simulink model "sim_cv3"  (R2019b)
settings: Solver=FixedStepAuto  StartTime=0.0  StopTime=1040  FixedStep=1  RelTol=1e-3
values from neighbouring files (symbols this model uses):
  AG = 0.95    [identifikacia_simulatora.m]    (also in identifikacia_simulatora2.m; simulator.m)
  G_INIT = 153    [cv5.m]    (also in identifikacia_simulatora.m = 158.4; identifikacia_simulatora2.m; simulator.m)
  GB = G_INIT    (= 158.4)    [identifikacia_simulatora.m]    (also in identifikacia_simulatora2.m = 153; simulator.m = 153)
  kI = ki    (= 0.1645)    [identifikacia_simulatora.m]    (also in identifikacia_simulatora2.m = 0.1939; simulator.m)
  p2 = 0.0106    [cv5.m]    (also in identifikacia_simulatora.m; identifikacia_simulatora2.m = 0.0097; simulator.m)
  p3 = p2    (= 0.0097)    [identifikacia_simulatora2.m]
  SG = S_G    (= 0.032)    [identifikacia_simulatora.m]    (also in identifikacia_simulatora2.m = 0.0159; simulator.m)
  SI = S_I    (= 0.00159)    [identifikacia_simulatora.m]    (also in identifikacia_simulatora2.m = 0.0014; simulator.m)
  TD = 33.474    [identifikacia_simulatora.m]    (also in identifikacia_simulatora2.m = 41.1727; simulator.m)
  TI = 44.55    [cv5.m]    (also in identifikacia_simulatora.m; identifikacia_simulatora2.m = 42.8216; simulator.m)
  VG = V_G    (= 1.467)    [identifikacia_simulatora.m]    (also in identifikacia_simulatora2.m; simulator.m)
  VI = 138.8    [cv5.m]    (also in identifikacia_simulatora.m; identifikacia_simulatora2.m = 110.599; simulator.m)
undefined symbols (not defined in the file or in its folder): p22, sigbuilder_block
settings Model: Creator=Miroslava  LastModifiedBy=shneeder
settings DataIOCC: ReturnWorkspaceOutputs=off
settings DebuggingCC: ArithmeticOperatorsInVariantConditions=warning
settings SFSimCC: SimUseLocalCustomCode=off  CustomCodeUndefinedFunction=UseInterfaceOnly
settings RTWCC: RTWUseLocalCustomCode=off

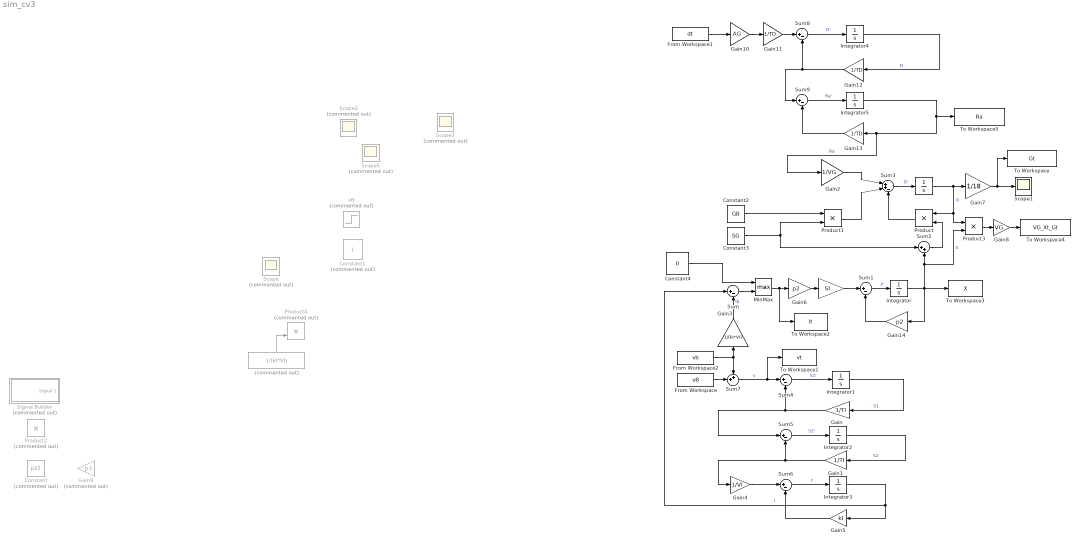
== system sim_cv3 ==
  " " : Gain  Gain=SI
  "   " : Integrator  InitialCondition=G_INIT
  " " : Constant  Commented=on  Value=1/(kI*VI)
  Constant : Constant  Commented=on  Value=p22
  Constant1 : Constant  Commented=on
  Constant2 : Constant  Value=GB
  Constant3 : Constant  Value=SG
  Constant4 : Constant  Value=0
  From Workspace : FromWorkspace  VariableName=vB  SampleTime=0
  From Workspace1 : FromWorkspace  VariableName=dt  SampleTime=0
  From Workspace2 : FromWorkspace  VariableName=vb  SampleTime=0
  Gain : Gain  Gain=1/TI
  Gain1 : Gain  Gain=1/TI
  Gain10 : Gain  Gain=AG
  Gain11 : Gain  Gain=1/TD
  Gain12 : Gain  Gain=1/TD
  Gain13 : Gain  Gain=1/TD
  Gain14 : Gain  Gain=p2
  Gain2 : Gain  Gain=1/VG
  Gain3 : Gain  Gain=1/(kI*VI)
  Gain4 : Gain  Gain=1/VI
  Gain5 : Gain  Gain=kI
  Gain6 : Gain  Gain=p2
  Gain7 : Gain  Gain=1/18
  Gain8 : Gain  Gain=VG
  Gain9 : Gain  Commented=on  Gain=p3
  Integrator{,1..2,4..5} (5 alike) : Integrator
  Integrator3 : Integrator  InitialCondition=6.5
  MinMax : MinMax  Function=max  Inputs=2
  Product : Product
  Product1 : Product
  Product2 : Product  Commented=on
  Product3 : Product
  Product4 : Product  Commented=on
  Scope{,2..3,5} (4 alike) : Scope  Commented=on
  Scope1 : Scope
  Signal Builder : Subsystem  Tag=STV Subsys  Commented=on  LoadFcn=sigbuilder_block('load');  StartFcn=sigbuilder_block('start');  StopFcn=sigbuilder_block('stop');  ClipboardFcn=sigbuilder_block('clipboard');  mask(Sigbuilder block){tuvar=[0:10]}
      mask help: Simulink:masks:SigbuilderBlock_MD
      mask init:
      | if ~strcmp(get_param(bdroot(gcbh),'SimulationStatus'),'stopped') tuvar = sigbuilder_block('maskInit'); end
      settings: CopyFcn=sigbuilder_block('copy');  DeleteFcn=sigbuilder_block('delete');  ModelCloseFcn=sigbuilder_block('modelClose');  PreSaveFcn=sigbuilder_block('preSave');  PauseFcn=sigbuilder_block('pause');  ContinueFcn=sigbuilder_block('continue');  NameChangeFcn=sigbuilder_block('namechange');  OpenFcn=sigbuilder_block('open',[429.75 192 565.5 389.25 ]);  CloseFcn=sigbuilder_block('close');
      mask Display: plot(0, 0, 100, 100,[2, 2, 32, 32, 2], [68, 8, 8, 68, 68],[32, 2], [38, 38], [32, 19, 2],[53, 60, 44], [32, 17, 17, 2],[16, 16, 31, 31]);txt = getActiveGroup(gcbh);text(2, 100, txt,'verticalAlignment', 'top');
  Sum{,1,4..6,8..9} (7 alike) : Sum  Inputs=|+-
  Sum2 : Sum  Inputs=|++
  Sum3 : Sum  Inputs=|++-
  Sum7 : Sum  Inputs=++|
  To Workspace : ToWorkspace  VariableName=Gt  SampleTime=-1
  To Workspace1 : ToWorkspace  VariableName=vt  SampleTime=-1
      settings: Save2DSignal=2-D array (concatenate along first dimension)
  To Workspace2 : ToWorkspace  VariableName=It  SampleTime=-1
      settings: Save2DSignal=2-D array (concatenate along first dimension)
  To Workspace3 : ToWorkspace  VariableName=X  SampleTime=-1
      settings: Save2DSignal=2-D array (concatenate along first dimension)
  To Workspace4 : ToWorkspace  VariableName=VG_Xt_Gt  SampleTime=-1
  To Workspace5 : ToWorkspace  VariableName=Ra  SaveFormat=Timeseries  SampleTime=-1
  vB : Step  Commented=on  Time=5  Before=40000  After=0  SampleTime=0
  wires:
  Integrator/1 -> To Workspace3/1, Gain14/1, Product3/2, Sum2/2  "X"
  Sum1/1 -> Integrator/1  "X'"
  Sum3/1 -> "   "/1  "G'"
  Constant2/1 -> Product1/1
  " "/1 -> Sum1/1
  Gain4/1 -> Sum6/1
  Sum4/1 -> Integrator1/1  "S1'"
  Sum7/1 -> To Workspace1/1, Sum4/1  "v"
  Sum6/1 -> Integrator3/1  "I'"
  Integrator1/1 -> Gain/1  "S1"
  Integrator3/1 -> Gain5/1, Sum/1  "I"
  Sum5/1 -> Integrator2/1  "S2'"
  Gain5/1 -> Sum6/2
  Integrator2/1 -> Gain1/1  "S2"
  Gain1/1 -> Gain4/1, Sum5/2
  "   "/1 -> Gain7/1, Product3/1, Product/1  "G"
  Sum2/1 -> Product/2
  Constant3/1 -> Product1/2, Sum2/1
  Gain2/1 -> Sum3/1
  Product/1 -> Sum3/3
  Product1/1 -> Sum3/2
  Gain6/1 -> " "/1
  Product3/1 -> Gain8/1
  Gain8/1 -> To Workspace4/1
  " "/1 -> Product4/2
  Gain7/1 -> Scope1/1, To Workspace/1
  From Workspace1/1 -> Gain10/1
  Gain10/1 -> Gain11/1
  Gain/1 -> Sum5/1, Sum4/2
  Gain11/1 -> Sum8/1
  Sum8/1 -> Integrator4/1  "D'"
  Integrator4/1 -> Gain12/1  "D"
  Gain12/1 -> Sum8/2, Sum9/1
  Sum9/1 -> Integrator5/1  "Ra'"
  Integrator5/1 -> To Workspace5/1, Gain13/1, Gain2/1  "Ra"
  Gain13/1 -> Sum9/2
  From Workspace2/1 -> Sum7/1, Gain3/1
  From Workspace/1 -> Sum7/2
  Gain14/1 -> Sum1/2
  Gain3/1 -> Sum/2  "Ib"
  Constant4/1 -> MinMax/1
  MinMax/1 -> To Workspace2/1, Gain6/1
  Sum/1 -> MinMax/2

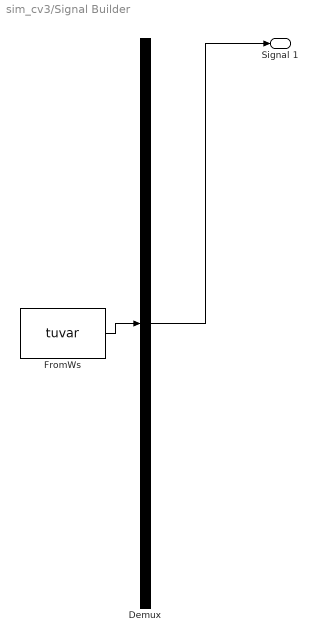
== system sim_cv3/Signal Builder ==
  Demux : Demux  Tag=STV Demux  Outputs=1
  FromWs : FromWorkspace  Tag=STV FromWs  VariableName=tuvar  SampleTime=0
      SigBuilderData=|
      | common.afterFinalStr = 'Extrapolate'
      | common.sampleTime = 0
      | dataSet.timeRange = [0 600]
      | dataSet.name = 'Group 1'
      | sbobj.Groups.Name = 'Group 1'
      | sbobj.Groups.Signals.Name = 'Signal 1'
      | sbobj.Groups.Signals.XData = [0 5 5 600]
      | sbobj.Groups.Signals.YData = [40000 40000 0 0]
      | sbobj.Groups.TimeRange = [0 600]
  Signal 1 : Outport  Tag=STV Outport
  wires:
  Demux/1 -> Signal 1/1
  FromWs/1 -> Demux/1
